simulink model "Sim"  (R2023b)
settings: Solver=VariableStepAuto  StartTime=0.0  StopTime=10.0  RelTol=1e-3
libraries: simrfV2elements x1, simulink x1
settings Model: Creator=megan  LastModifiedBy=megan

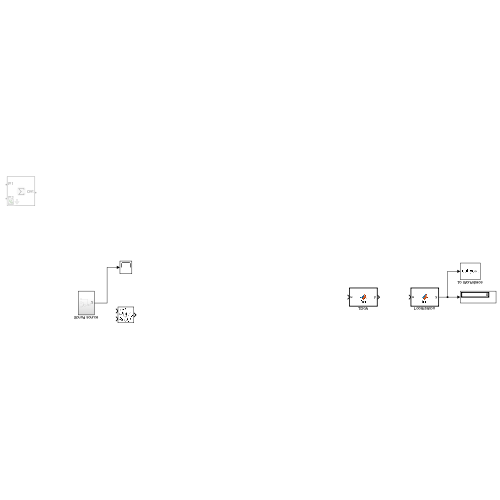
[thumbnail: Simulink's stored preview of the top-level diagram]
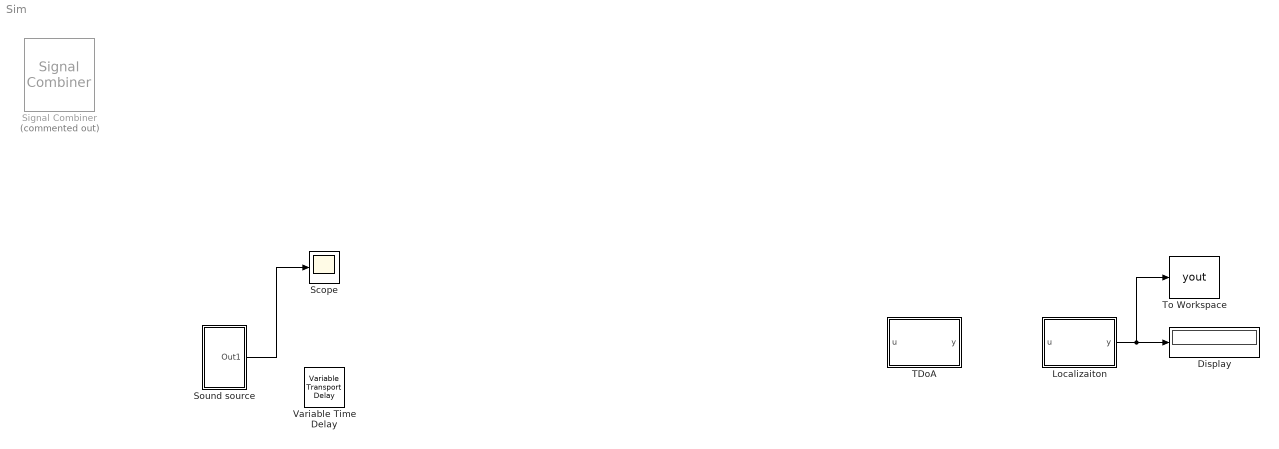
== system Sim ==
  Display : Display
  Localizaiton : MATLAB Function  TreatAsAtomicUnit=on
  Scope : Scope
  Signal Combiner : simrfV2elements/Signal Combiner  Commented=on  classname=signal_sum_mask  InternalGrounding=on
  Sound source : Subsystem
  TDoA : MATLAB Function  TreatAsAtomicUnit=on
  To Workspace : ToWorkspace  VariableName=yout  SampleTime=-1
      settings: Save2DSignal=2-D array (concatenate along first dimension)
  Variable Time Delay : VariableTransportDelay  MaximumDelay=10
  wires:
  Sound source/1(Out1) -> Scope/1
  Localizaiton/1(y) -> To Workspace/1, Display/1

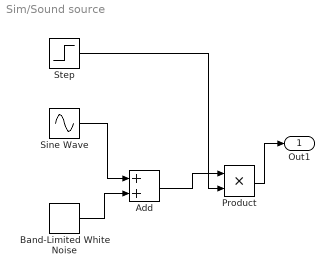
== system Sim/Sound source ==
  Add : Sum
  Band-Limited White Noise : simulink/Sources/Band-Limited White Noise  Cov=[0.1]  Ts=0.1  seed=[23341]
  Product : Product
  Sine Wave : Sin  SampleTime=0
  Step : Step  Time=5  Before=1  After=0  SampleTime=0
  Out1 : Outport
  wires:
  Band-Limited White Noise/1 -> Add/2
  Sine Wave/1 -> Add/1
  Step/1 -> Product/2
  Product/1 -> Out1/1
  Add/1 -> Product/1

== matlab function Sim/Localizaiton ==
  data: u input; y output
function y = fcn(u)

y = u;

== matlab function Sim/TDoA ==
  data: u input; y output
function y = fcn(u)

y = u;
